simulink model "COMPARE_AVG_TB"  (R2024a)
settings: Solver=VariableStepAuto  StartTime=0.0  StopTime=2000  RelTol=1e-3
PreLoadFcn:
  | N = 100;
InitFcn:
  | N = 100;
libraries: dspstat3 x5, simulink x2, dspsrcs4 x1
settings Model: Creator=kschutz  LastModifiedBy=kschutz

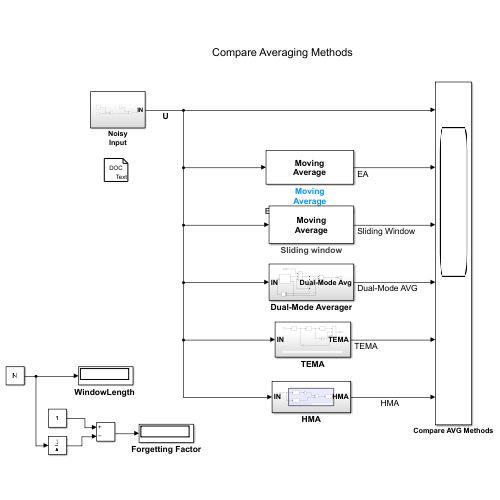
[thumbnail: Simulink's stored preview of the top-level diagram]
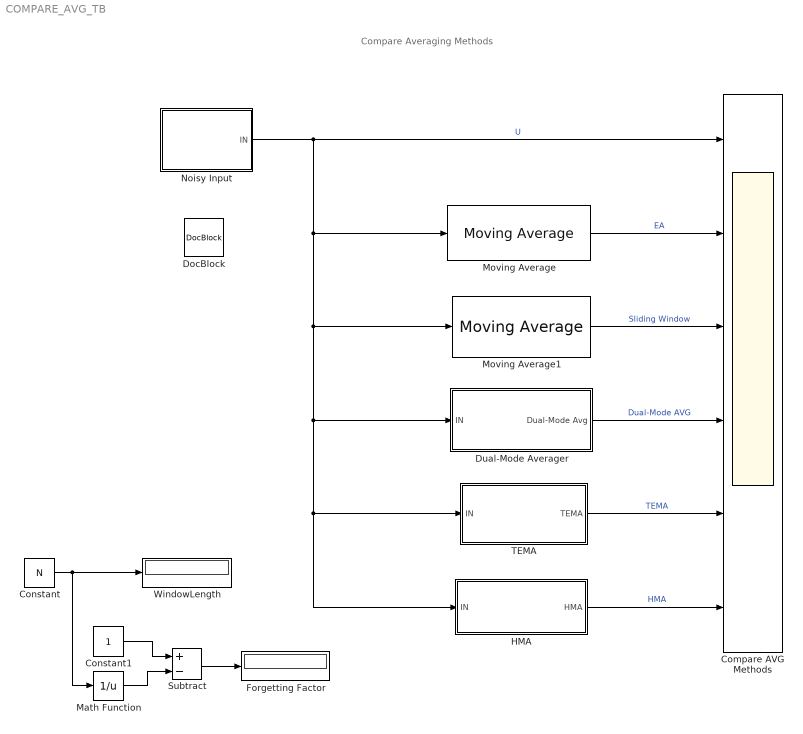
== system COMPARE_AVG_TB ==
  note: Compare Averaging Methods
  Compare AVG Methods : Scope  NumInputPorts=6
  Constant : Constant  Value=N
  Constant1 : Constant
  DocBlock : simulink/Model-Wide Utilities/DocBlock  DocumentType=Text
      content=|
      | One could attempt to get the best of both worlds and
      | dynamically tune the averaging coefficients in the
      | sliding and exponential averagers by constantly looking
      | at the rate of change of the mean.
      |
      | If the rate of change of the mean exceeded a threshold in
      | the case of the sliding window, one could use a smaller N.
      | In the case of the exponential averager, one could reset
      | the exponential weights and allow them to converge again,
      | like at startup.
  Dual-Mode Averager : Subsystem
  Forgetting Factor : Display
  HMA : Subsystem
  Math Function : Math  Operator=reciprocal
  Moving Average : dspstat3/Moving Average  Method=Exponential weighting  ForgettingFactorPort=off  SpecifyWindowLength=on  WindowLength=N  OverlapLength=15  AllowArbitraryInputLength=off  ForgettingFactor=1-1/N  SimulateUsing=Code generation
      settings: AttributesFormatString=%<Method>
  Moving Average1 : dspstat3/Moving Average  Method=Sliding window  ForgettingFactorPort=off  SpecifyWindowLength=on  WindowLength=N  OverlapLength=N-1  AllowArbitraryInputLength=off  ForgettingFactor=1  SimulateUsing=Code generation
      settings: AttributesFormatString=%<Method>
  Noisy Input : Subsystem
  Subtract : Sum  Inputs=+-
  TEMA : Subsystem
  "WindowLength " : Display
  wires:
  Noisy Input/1(IN) -> Moving Average/1, Dual-Mode Averager/1(IN), TEMA/1(IN), HMA/1(IN), Moving Average1/1, Compare AVG Methods/1  "U"
  Moving Average/1 -> Compare AVG Methods/2  "EA"
  Moving Average1/1 -> Compare AVG Methods/3  "Sliding Window"
  Dual-Mode Averager/1(Dual-Mode Avg) -> Compare AVG Methods/4  "Dual-Mode AVG"
  TEMA/1(TEMA) -> Compare AVG Methods/5  "TEMA"
  HMA/1(HMA) -> Compare AVG Methods/6  "HMA"
  Constant/1 -> Math Function/1, "WindowLength "/1
  Math Function/1 -> Subtract/2
  Constant1/1 -> Subtract/1
  Subtract/1 -> Forgetting Factor/1

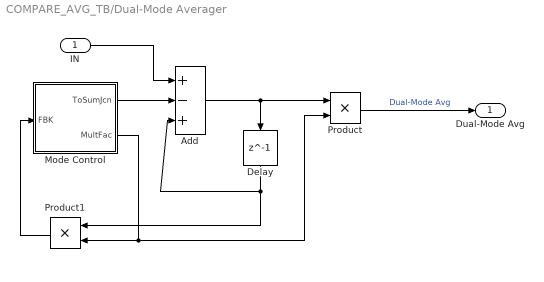
== system COMPARE_AVG_TB/Dual-Mode Averager ==
  IN : Inport
  Add : Sum  Inputs=+-+
  Delay : Delay  DelayLength=1
  Mode Control : Subsystem
  Product : Product
  Product1 : Product
  Dual-Mode Avg : Outport  VectorParamsAs1DForOutWhenUnconnected=off
  wires:
  Add/1 -> Product/1, Delay/1
  Mode Control/2(MultFac) -> Product1/2, Product/2
  Delay/1 -> Product1/1, Add/3
  Mode Control/1(ToSumJcn) -> Add/2
  Product/1 -> Dual-Mode Avg/1  "Dual-Mode Avg"
  IN/1 -> Add/1
  Product1/1 -> Mode Control/1(FBK)

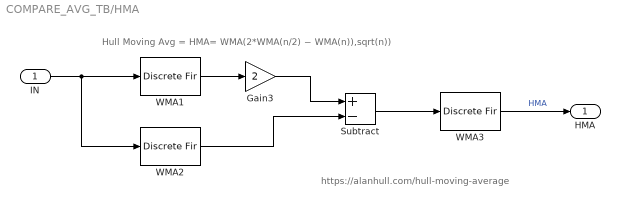
== system COMPARE_AVG_TB/HMA ==
  note: Hull Moving Avg = HMA= WMA(2*WMA(n/2) − WMA(n)),sqrt(n))
  note: https://alanhull.com/hull-moving-average
  IN : Inport
  Gain3 : Gain  Gain=2
  Subtract : Sum  Inputs=+-
  WMA1 : DiscreteFir  Coefficients=[N/2:-1:1]/sum(1:N/2)
  WMA2 : DiscreteFir  Coefficients=[N:-1:1]/sum(1:N)
  WMA3 : DiscreteFir  Coefficients=[sqrt(N):-1:1]/sum(1:sqrt(N))
  HMA : Outport
  wires:
  WMA3/1 -> HMA/1  "HMA"
  WMA1/1 -> Gain3/1
  Gain3/1 -> Subtract/1
  IN/1 -> WMA1/1, WMA2/1
  WMA2/1 -> Subtract/2
  Subtract/1 -> WMA3/1

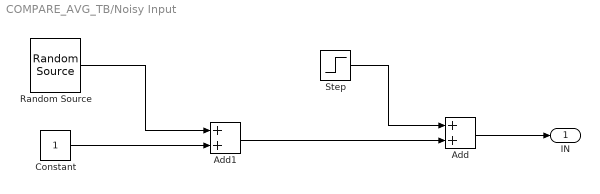
== system COMPARE_AVG_TB/Noisy Input ==
  Add : Sum
  Add1 : Sum
  Constant : Constant  SampleTime=1
  Random Source : dspsrcs4/Random Source  SrcType=Gaussian  MinVal=0  MaxVal=1  MeanVal=0  VarVal=.2  RepMode=Specify seed  rawSeed=123  IsInherit=off  SampTime=1  SampFrame=1  OutComplex=Real  DataType=double  SimulateUsing=Interpreted execution
  Step : Step  Time=500  SampleTime=0
  IN : Outport  VectorParamsAs1DForOutWhenUnconnected=off
  wires:
  Constant/1 -> Add1/2
  Random Source/1 -> Add1/1
  Add/1 -> IN/1
  Add1/1 -> Add/2
  Step/1 -> Add/1

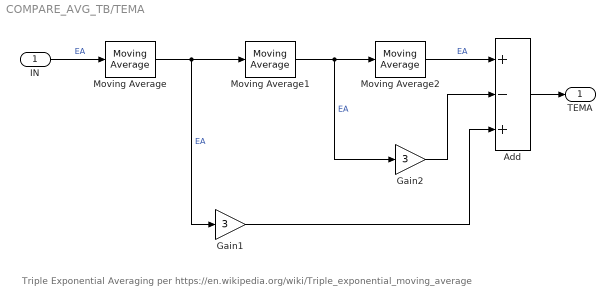
== system COMPARE_AVG_TB/TEMA ==
  note: Triple Exponential Averaging per https://en.wikipedia.org/wiki/Triple_exponential_moving_average
  IN : Inport
  Add : Sum  Inputs=+-+
  Gain1 : Gain  Gain=3
  Gain2 : Gain  Gain=3
  Moving Average : dspstat3/Moving Average  Method=Exponential weighting  ForgettingFactorPort=off  SpecifyWindowLength=on  WindowLength=20  OverlapLength=19  AllowArbitraryInputLength=off  ForgettingFactor=(N-1)/N  SimulateUsing=Interpreted execution
      settings: AttributesFormatString=FF = %<ForgettingFactor>
  Moving Average1 : dspstat3/Moving Average  Method=Exponential weighting  ForgettingFactorPort=off  SpecifyWindowLength=on  WindowLength=20  OverlapLength=19  AllowArbitraryInputLength=off  ForgettingFactor=(N-1)/N  SimulateUsing=Interpreted execution
      settings: AttributesFormatString=FF = %<ForgettingFactor>
  Moving Average2 : dspstat3/Moving Average  Method=Exponential weighting  ForgettingFactorPort=off  SpecifyWindowLength=on  WindowLength=20  OverlapLength=19  AllowArbitraryInputLength=off  ForgettingFactor=(N-1)/N  SimulateUsing=Interpreted execution
      settings: AttributesFormatString=FF = %<ForgettingFactor>
  TEMA : Outport
  wires:
  Moving Average/1 -> Gain1/1, Moving Average1/1  "EA"
  Moving Average2/1 -> Add/1  "EA"
  Gain2/1 -> Add/2
  Gain1/1 -> Add/3
  IN/1 -> Moving Average/1  "EA"
  Moving Average1/1 -> Gain2/1, Moving Average2/1  "EA"
  Add/1 -> TEMA/1

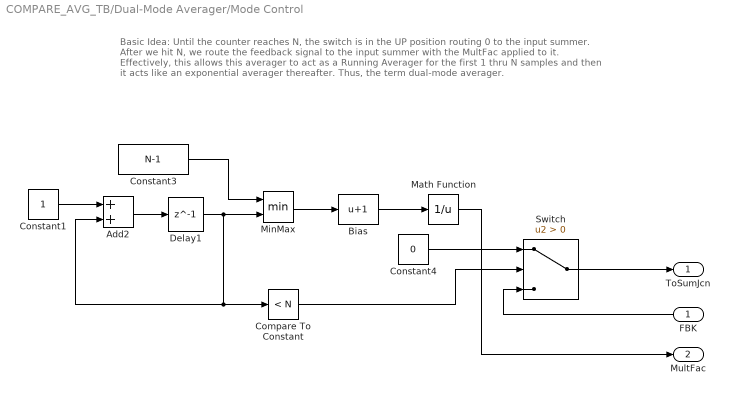
== system COMPARE_AVG_TB/Dual-Mode Averager/Mode Control ==
  note: Basic Idea: Until the counter reaches N, the switch is in the UP position routing 0 to the input summer.
      | After we hit N, we route the feedback signal to the input summer with the MultFac applied to it.
      | Effectively, this allows this averager to act as a Running Averager for the first 1 thru N samples
      | and then it acts like an exponential averager thereafter. Thus, the term dual-mode averager.
  FBK : Inport
  Add2 : Sum
  Bias : Bias  Bias=1  SaturateOnIntegerOverflow=off
  Compare To Constant : simulink/Logic and Bit Operations/Compare To Constant  relop=<  const=N  OutDataTypeStr=boolean
  Constant1 : Constant
  Constant3 : Constant  Value=N-1  OutDataTypeStr=single  SampleTime=1
  Constant4 : Constant  Value=0
  Delay1 : Delay  DelayLength=1  InitialCondition=0
  Math Function : Math  Operator=reciprocal  SignedPower=on
  MinMax : MinMax  Inputs=2
  Switch : Switch  Criteria=u2 > Threshold  SaturateOnIntegerOverflow=off  InputSameDT=off
  ToSumJcn : Outport  VectorParamsAs1DForOutWhenUnconnected=off
  MultFac : Outport  Port=2  VectorParamsAs1DForOutWhenUnconnected=off
  wires:
  Delay1/1 -> MinMax/2, Compare To Constant/1, Add2/2
  Switch/1 -> ToSumJcn/1
  Add2/1 -> Delay1/1
  Constant1/1 -> Add2/1
  Bias/1 -> Math Function/1
  MinMax/1 -> Bias/1
  Constant4/1 -> Switch/1
  Constant3/1 -> MinMax/1
  Compare To Constant/1 -> Switch/2
  FBK/1 -> Switch/3
  Math Function/1 -> MultFac/1
